simulink model "Adaptive"  (R2022b)
settings: Solver=VariableStepAuto  StartTime=0.0  StopTime=50  RelTol=1e-3
values from neighbouring files (symbols this model uses):
  A_sys = [0,1;-a0_sys,-a1_sys]    [constants.m]
  Am = [0,1;-am0,-am1]    [constants.m]
  b_sys = [0;b0_sys]    [constants.m]
  bm = [0;am0]    [constants.m]
  cm = [1,0]    [constants.m]
  k = b0/am0    (= 0.00117685479671)    [constants.m]
  lambda = 100    [constants.m]
  P = [double(sol.P1_1), double(sol.P1_2) ... (first row only)    [constants.m]
  theta = [theta1,theta2]'    [constants.m]
  Theta = [(-am0+a0_sys)/b0; (-am1+a1_sys)/b0]    [constants.m]
settings Model: Creator=zein  LastModifiedBy=zein

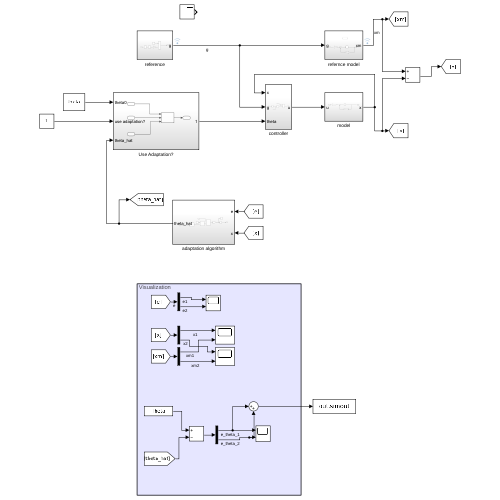
[thumbnail: Simulink's stored preview of the top-level diagram]
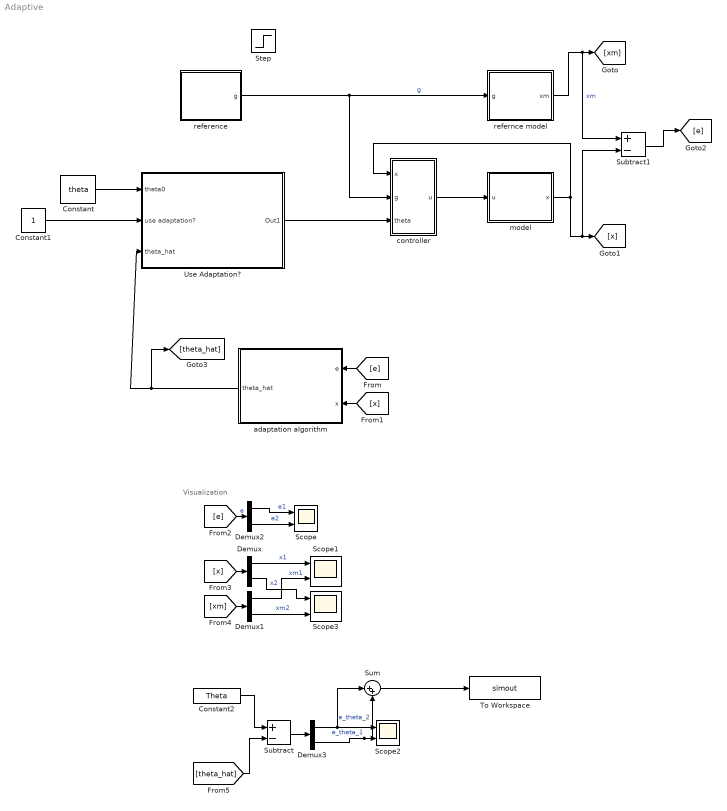
== system Adaptive ==
  note: Visualization
  Constant : Constant  Value=theta  VectorParams1D=off
  Constant1 : Constant
  Constant2 : Constant  Value=Theta
  Demux{,1..3} (4 alike) : Demux  Outputs=2
  Scope{,1..3} (4 alike) : Scope  NumInputPorts=2
  Step : Step  Time=0  SampleTime=0
  Subtract : Sum  Inputs=+-
  Subtract1 : Sum  Inputs=+-
  Sum : Sum  Inputs=|++
  To Workspace : ToWorkspace  VariableName=simout  SaveFormat=Timeseries  SampleTime=-1
  Use Adaptation? : Subsystem
  adaptation algorithm : Subsystem
  controller : Subsystem
  model : Subsystem
  reference : Subsystem
  refernce model : Subsystem
  wires:
  reference/1(g) -> controller/2(g), refernce model/1(g)  "g"
  refernce model/1(xm) -> Subtract1/1, [xm]  "xm"
  controller/1(u) -> model/1(u)
  Constant/1 -> Use Adaptation?/1(theta0)
  Constant1/1 -> Use Adaptation?/2(use adaptation?)
  adaptation algorithm/1(theta_hat) -> [theta_hat], Use Adaptation?/3(theta_hat)
  Use Adaptation?/1(Out1) -> controller/3(theta)
  Subtract1/1 -> [e]
  [e] -> adaptation algorithm/1(e)
  [x] -> adaptation algorithm/2(x)
  [e] -> Demux2/1  "e"
  Constant2/1 -> Subtract/1
  [theta_hat] -> Subtract/2
  Subtract/1 -> Demux3/1
  [x] -> Demux/1
  [xm] -> Demux1/1
  Demux/1 -> Scope1/1  "x1"
  Demux/2 -> Scope3/1  "x2"
  Demux1/1 -> Scope1/2  "xm1"
  Demux1/2 -> Scope3/2  "xm2"
  model/1(x) -> controller/1(x), Subtract1/2, [x]
  Demux2/1 -> Scope/1  "e1"
  Demux2/2 -> Scope/2  "e2"
  Demux3/1 -> Sum/1, Scope2/1  "e_theta_1"
  Demux3/2 -> Sum/2, Scope2/2  "e_theta_2"
  Sum/1 -> To Workspace/1

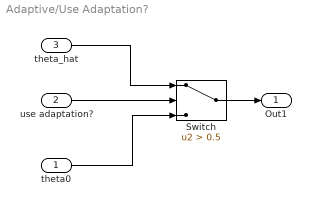
== system Adaptive/Use Adaptation? ==
  theta0 : Inport
  use adaptation? : Inport  Port=2
  theta_hat : Inport  Port=3
  Switch : Switch  Criteria=u2 > Threshold  Threshold=0.5  SaturateOnIntegerOverflow=off  InputSameDT=off
  Out1 : Outport
  wires:
  use adaptation?/1 -> Switch/2
  theta_hat/1 -> Switch/1
  theta0/1 -> Switch/3
  Switch/1 -> Out1/1

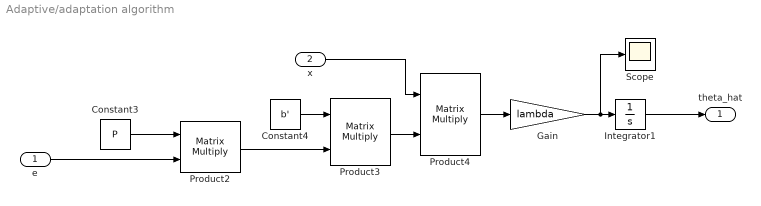
== system Adaptive/adaptation algorithm ==
  e : Inport
  x : Inport  Port=2
  Constant3 : Constant  Value=P  VectorParams1D=off
  Constant4 : Constant  Value=b'  VectorParams1D=off
  Gain : Gain  Gain=lambda
  Integrator1 : Integrator  InitialCondition=[0;0]
  Product2 : Product  Multiplication=Matrix(*)
  Product3 : Product  Multiplication=Matrix(*)
  Product4 : Product  Multiplication=Matrix(*)
  Scope : Scope
  theta_hat : Outport
  wires:
  Product2/1 -> Product3/2
  Product3/1 -> Product4/2
  Product4/1 -> Gain/1
  Constant4/1 -> Product3/1
  Gain/1 -> Scope/1, Integrator1/1
  e/1 -> Product2/2
  Integrator1/1 -> theta_hat/1
  Constant3/1 -> Product2/1
  x/1 -> Product4/1

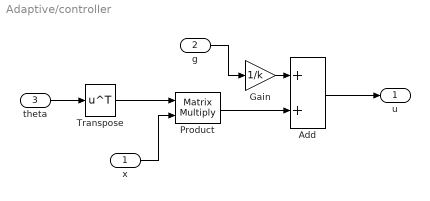
== system Adaptive/controller ==
  x : Inport
  g : Inport  Port=2
  theta : Inport  Port=3
  Add : Sum
  Gain : Gain  Gain=1/k
  Product : Product  Multiplication=Matrix(*)
  Transpose : Math  Operator=transpose
  u : Outport
  wires:
  g/1 -> Gain/1
  Product/1 -> Add/2
  x/1 -> Product/2
  Add/1 -> u/1
  Gain/1 -> Add/1
  theta/1 -> Transpose/1
  Transpose/1 -> Product/1

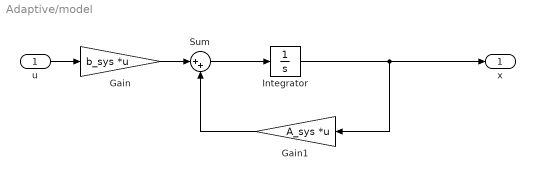
== system Adaptive/model ==
  u : Inport
  Gain : Gain  Gain=b_sys  Multiplication=Matrix(K*u)
  Gain1 : Gain  Gain=A_sys  Multiplication=Matrix(K*u)
  Integrator : Integrator  InitialCondition=[0;0]
  Sum : Sum  Inputs=|++
  x : Outport
  wires:
  u/1 -> Gain/1
  Integrator/1 -> x/1, Gain1/1
  Sum/1 -> Integrator/1
  Gain1/1 -> Sum/2
  Gain/1 -> Sum/1

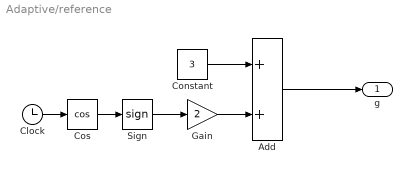
== system Adaptive/reference ==
  Add : Sum
  Clock : Clock
  Constant : Constant  Value=3
  Cos : Trigonometry  Operator=cos
  Gain : Gain  Gain=2
  Sign : Signum
  g : Outport
  wires:
  Clock/1 -> Cos/1
  Sign/1 -> Gain/1
  Constant/1 -> Add/1
  Add/1 -> g/1
  Cos/1 -> Sign/1
  Gain/1 -> Add/2

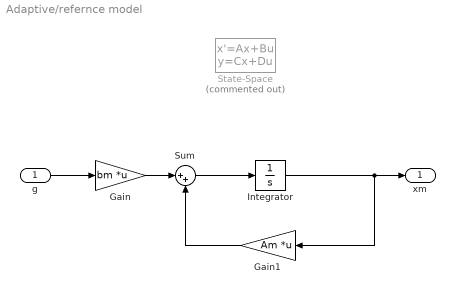
== system Adaptive/refernce model ==
  g : Inport
  Gain : Gain  Gain=bm  Multiplication=Matrix(K*u)
  Gain1 : Gain  Gain=Am  Multiplication=Matrix(K*u)
  Integrator : Integrator  InitialCondition=[0;0]
  State-Space : StateSpace  Commented=on  A=Am  B=bm  C=cm  D=0  InitialCondition=0
  Sum : Sum  Inputs=|++
  xm : Outport
  wires:
  Integrator/1 -> Gain1/1, xm/1
  g/1 -> Gain/1
  Gain/1 -> Sum/1
  Gain1/1 -> Sum/2
  Sum/1 -> Integrator/1
